simulink model "t1"  (R2016a)
settings: Solver=VariableStepAuto  SolverMode=SingleTasking  StartTime=0.0  StopTime=10.0  RelTol=1e-3
settings Model: Creator=admin  LastModifiedBy=admin
settings DataIOCC: LimitDataPoints=on  SaveOutput=off  SaveTime=off
settings OptimizationCC: BlockReduction=off  BooleanDataType=off
settings DebuggingCC: SaveWithParameterizedLinksMsg=none  UnderspecifiedInitializationDetection=Classic  MergeDetectMultiDrivingBlocksExec=none  SignalResolutionControl=TryResolveAllWithWarning  AllowSymbolicDim=off
settings HardwareCC: TargetUnknown=on

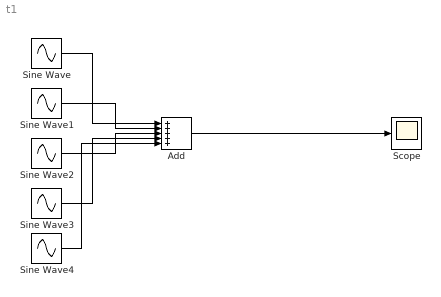
== system t1 ==
  Add : Sum  Inputs=+++++
  Scope : Scope
  Sine Wave : Sin  Frequency=2*pi  SampleTime=0
  Sine Wave1 : Sin  Amplitude=1/3  Frequency=3*2*pi  SampleTime=0
  Sine Wave2 : Sin  Amplitude=1/5  Frequency=5*2*pi  SampleTime=0
  Sine Wave3 : Sin  Amplitude=1/7  Frequency=7*2*pi  SampleTime=0
  Sine Wave4 : Sin  Amplitude=1/9  Frequency=9*2*pi  SampleTime=0
  wires:
  Sine Wave/1 -> Add/1
  Sine Wave1/1 -> Add/2
  Sine Wave2/1 -> Add/3
  Sine Wave3/1 -> Add/4
  Sine Wave4/1 -> Add/5
  Add/1 -> Scope/1
